simulink model "P5_Ex20"  (R2018a)
settings: Solver=FixedStepAuto  StartTime=0.0  StopTime=20  RelTol=1e-3  EnableMultiTasking=on
PreLoadFcn:
  |     K0=0.82/0.017;
  |     tau0=0.26;
  |     % modelització del sistema a partir de les seves característiques
  |     N=9;
  |     Kpot=1.62;
  |     planta=tf([K0],[tau0 1]);
  |     conversor=tf([1],[N 0]);
  |     potenciometre=tf([Kpot],[1]);
  | 
  |     % modelització en temps continu
  |     sistema_continu=planta*conversor*potenciometre;
  |     Ts=0.005;
  |     Tg=0.005;
  |     zc=1;
  |     zp=1;
  |     k=1;
  |     Total_time=20;
  |     % repeticions
  |     N=2.5;
  |     T_ona=Total_time/N;
  |     Ts_dif=1.0000e-003;
  |     Ts=0.01;
  |     i=1;
  |     Vmax=3;
  |     Vmin=-3;
  |     input_vector=[Vmax Vmin];
  |     while (i<=N)
  |         input_vector=[input_vector [Vmax Vmin]];
  |         i=i+1;
  |     end
libraries: arduinolib x4, simulink x2
settings Model: SimulationMode=external  ExtModeTrigDuration=2  Creator=Eneko Lerma  LastModifiedBy=Eneko Lerma
settings SolverCC: AutoInsertRateTranBlk=on
settings OptimizationCC: EnhancedBackFolding=on  PassReuseOutputArgsAs=Individual arguments  MaxStackSize=64  OptimizeBlockOrder=speed  DifferentSizesBufferReuse=on  OptimizationCustomize=off
settings DebuggingCC: ParameterTunabilityLossMsg=error
settings HardwareCC: ProdBitPerPointer=32  ProdBitPerSizeT=32  ProdBitPerPtrDiffT=32  ProdLargestAtomicInteger=Long  ProdLargestAtomicFloat=Double  ProdWordSize=32  ProdHWDeviceType=ARM Compatible->ARM Cortex
settings SFSimCC: MATLABDynamicMemAlloc=off
settings RTWCC: SystemTargetFile=ert.tlc  HardwareBoard=Arduino Due  TLCOptions=-aInlineSetEventsForThisBaseRateFcn=TLC_FALSE -aSuppressMultiTaskScheduler=TLC_FALSE -aRateBasedStepFcn=1  TemplateMakefile=ert_default_tmf  GenerateReport=on  Toolchain=Arduino ARM  BuildConfiguration=Faster Runs  IncludeHyperlinkInReport=on  LaunchReport=on  GenerateTraceInfo=on  GenerateTraceReport=on  GenerateTraceReportSl=on  GenerateTraceReportSf=on  GenerateTraceReportEml=on
settings RTWCC: CustomTerminator=|
  | writeDigitalPin((uint8_T)3, 0);
  | writeDigitalPin((uint8_T)5, 0);
settings CodeAppCC: ForceParamTrailComments=on  IgnoreCustomStorageClasses=off  OperatorAnnotations=on  SimulinkDataObjDesc=on  SFDataObjDesc=on  InsertBlockDesc=on
settings ERTTargetCC: SupportContinuousTime=on  SupportVariableSizeSignals=on

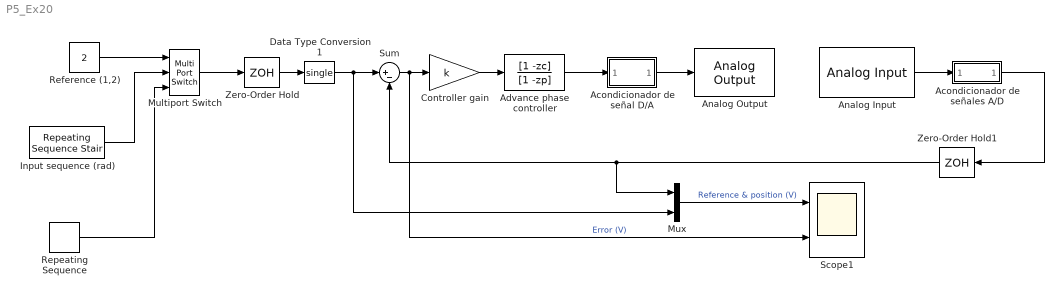
== system P5_Ex20 ==
  Acondicionador de señal D/A : Subsystem
  Acondicionador de señales A/D : Subsystem
  Advance phase controller : DiscreteTransferFcn  Numerator=[1 -zc]  Denominator=[1 -zp]  SampleTime=Ts
  Analog Input : arduinolib/Analog Input  pinNumber=1  ReadResultsOnly=off  ConversionTriggerSource=Software  ExternalTriggerType=uint32(0)  OutputDataType=uint16  EnableConversionCompleteNotify=off  EnableOuputStatus=off  SampleTime=0.005  blockPlatform=arduino
  Analog Output : arduinolib/Analog Output  DACpin=DAC1  blockPlatform=arduino
      settings: SourceProductName=Simulink Support Package for Arduino Hardware  SourceProductBaseCode=ARDUINO
  Controller gain : Gain  Gain=k
  Data Type Conversion1 : DataTypeConversion  OutDataTypeStr=single
  Input sequence (rad) : simulink/Sources/Repeating Sequence Stair  OutValues=input_vector  tsamp=T_ona/2  OutMin=[]  OutMax=[]  OutDataTypeStr=double  OutputDataTypeScalingMode=double  OutDataType=float('double')  ConRadixGroup=Best Precision: Vector-wise  OutScaling=2^-12
  Multiport Switch : MultiPortSwitch  Inputs=2
  Mux : Mux  Inputs=2
  Reference (1,2) : Constant  Value=2
  Repeating Sequence : simulink/Sources/Repeating Sequence  rep_seq_t="[0    0.1000    0.2000    0.3000    0.4000    0.5000    0.6000    0.7000    0.8000 0.9000    1.0000    1.1000    1.2000    1.3000    1.4000    1.5000    1.6000    1.7000 1.8000    1.9000    2.0000    2.1000    2.2000    2.3000    2.4000    2.5000    2.6000 2.7000    2.8000    2.9000    3.0000    3.1000    3.2000    3.3000    3.4000    3.5000\t3.6000    3.7000    3.8000    3.9000    4.0000    4.1000    4.2000    4.3000    4.4000    4.5000    4.6000    4.7000    4.8000    4.9000    5.0000]"  rep_seq_y=[-2.0000,-1.9200,-1.8400,-1.7600,-1.6800,-1.6000,-1.5200,-1.4400,-1.3600,-1.2800,-1.2000,-1.1200,-1.0400,-0.9600,-0.8800,-0.8000,-0.7200,-0.6400,-0.5600,-0.4800,-0.4000,-0.3200,-0.2400,-0.1600,-0.0800,0,0.0800,0.1600,0.2400,0.3200,0.4000,0.4800,0.5600,0.6400,0.7200,0.8000,0.8800,0.9600,1.0400,1.1200,1.2000,1.2800,1.3600,1.4400,1.5200,1.6000,1.6800,1.7600,1.8400,1.9200,2.0000]
  Scope1 : Scope  NumInputPorts=2
  Sum : Sum  Inputs=|+-
  Zero-Order Hold : ZeroOrderHold  SampleTime=Ts
  Zero-Order Hold1 : ZeroOrderHold  SampleTime=Ts
  wires:
  Reference (1,2)/1 -> Multiport Switch/1
  Sum/1 -> Scope1/2, Controller gain/1  "Error (V)"
  Repeating Sequence/1 -> Multiport Switch/3
  Mux/1 -> Scope1/1  "Reference & position (V)"
  Input sequence (rad)/1 -> Multiport Switch/2
  Controller gain/1 -> Advance phase controller/1
  Acondicionador de señales A/D/1(" ") -> Zero-Order Hold1/1
  Acondicionador de señal D/A/1(" ") -> Analog Output/1
  Advance phase controller/1 -> Acondicionador de señal D/A/1("  ")
  Zero-Order Hold/1 -> Data Type Conversion1/1
  Multiport Switch/1 -> Zero-Order Hold/1
  Zero-Order Hold1/1 -> Mux/1, Sum/2
  Analog Input/1 -> Acondicionador de señales A/D/1("  ")
  Data Type Conversion1/1 -> Mux/2, Sum/1

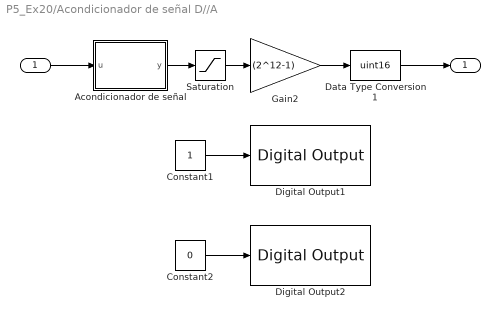
== system P5_Ex20/Acondicionador de señal D//A ==
  "  " : Inport  OutDataTypeStr=single
  Acondicionador de señal : MATLAB Function  TreatAsAtomicUnit=on
  Constant1 : Constant
  Constant2 : Constant  Value=0
  Data Type Conversion1 : DataTypeConversion  OutDataTypeStr=uint16
  Digital Output1 : arduinolib/Digital Output  pinNumber=5  blockPlatform=arduino
  Digital Output2 : arduinolib/Digital Output  pinNumber=3  blockPlatform=arduino
  Gain2 : Gain  Gain=(2^12-1)  OutDataTypeStr=single
  Saturation : Saturate  UpperLimit=1  LowerLimit=0  OutDataTypeStr=single
  " " : Outport  OutDataTypeStr=uint16
  wires:
  Gain2/1 -> Data Type Conversion1/1
  "  "/1 -> Acondicionador de señal/1(u)
  Acondicionador de señal/1(y) -> Saturation/1
  Data Type Conversion1/1 -> " "/1
  Saturation/1 -> Gain2/1
  Constant1/1 -> Digital Output1/1
  Constant2/1 -> Digital Output2/1

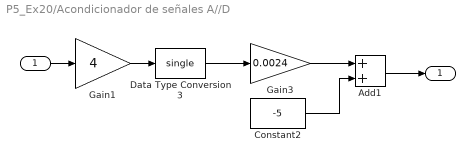
== system P5_Ex20/Acondicionador de señales A//D ==
  "  " : Inport  OutDataTypeStr=uint16
  Add1 : Sum  AccumDataTypeStr=single
  Constant2 : Constant  Value=-5  OutDataTypeStr=single  SampleTime=Ts
  Data Type Conversion3 : DataTypeConversion  OutDataTypeStr=single
  Gain1 : Gain  Gain=4  OutDataTypeStr=uint16
  Gain3 : Gain  Gain=0.0024  OutDataTypeStr=single
  " " : Outport  OutDataTypeStr=single
  wires:
  Gain1/1 -> Data Type Conversion3/1
  "  "/1 -> Gain1/1
  Data Type Conversion3/1 -> Gain3/1
  Gain3/1 -> Add1/1
  Constant2/1 -> Add1/2
  Add1/1 -> " "/1

== matlab function P5_Ex20/Acondicionador de señal D//A/Acondicionador de señal ==
  data: u input; y output
function y = fcn(u)
y =0.0968*u+0.5085;
